simulink model "model_T_PSH_IEEE39"  (R2020b)
settings: Solver=ode3  StartTime=0.0  StopTime=300  FixedStep=Ts  RelTol=1e-3
PostLoadFcn:
  | IEEE39BusLineLength;
  | vNomHV = 345E3;fNom=60;load('Dynamicload.mat');
InitFcn:
  | IEEE39BusLineLength;
  | vNomHV = 345E3;fNom=60;load('Dynamicload.mat');
values from neighbouring files (symbols this model uses):
  At = 1.48    [MAIN_T_PSH_IEEE39.m]
  Dturb = 0.3    [MAIN_T_PSH_IEEE39.m]
  fix_mode = 1    [MAIN_T_PSH_IEEE39.m]
  Gmax = 1    [MAIN_T_PSH_IEEE39.m]
  Gmin = 0    [MAIN_T_PSH_IEEE39.m]
  Hdam = 1    [MAIN_T_PSH_IEEE39.m]
  Kd = 1    [MAIN_T_PSH_IEEE39.m]    (also in plots_T_PSH_IEEE39.m)
  max_delay_gen2pump = 20    [MAIN_T_PSH_IEEE39.m]
  max_delay_pump2hsc = 30    [MAIN_T_PSH_IEEE39.m]
  pgen_pump = Kd*Pref    (= 0.9)    [MAIN_T_PSH_IEEE39.m]
  pgen_turb = (1-Kd)*Pref    (= 0)    [MAIN_T_PSH_IEEE39.m]
  pgen_turb_gen2pump = (1-kd_gen2pump)*Pref    (= 0)    [MAIN_T_PSH_IEEE39.m]
  pgen_turb_hsc2gen = (1-kd_hsc2gen)*Pref    (= 0.36)    [MAIN_T_PSH_IEEE39.m]
  pgen_turb_pump2hsc = (1-kd_pump2hsc)*Pref    (= 0.36)    [MAIN_T_PSH_IEEE39.m]
  Pref = 0.9    [MAIN_T_PSH_IEEE39.m]    (also in MAIN_VS_PSH.m = 1)
  qNL = 0.1    [MAIN_T_PSH_IEEE39.m]
  R = 0.04    [MAIN_T_PSH_IEEE39.m]
  r = 0.31    [MAIN_T_PSH_IEEE39.m]
  Rp = 0.05    [IEEE39BusLineLength.m]
  Sn = 320E6    (= 320000000)    [MAIN_T_PSH_IEEE39.m]
  t_gen2pump = 10    [MAIN_T_PSH_IEEE39.m]
  t_hsc2gen = 150    [MAIN_T_PSH_IEEE39.m]
  t_pump2hsc = 35    [MAIN_T_PSH_IEEE39.m]
  t_sw_off = 220    [MAIN_FS_PSH_IEEE39.m]    (also in MAIN_T_PSH_IEEE39.m; MAIN_VS_PSH.m = 45)
  t_sw_on = 130    [MAIN_FS_PSH_IEEE39.m]    (also in MAIN_T_PSH_IEEE39.m; MAIN_VS_PSH.m = 35)
  Tf = 0.05    [MAIN_T_PSH_IEEE39.m]
  Tg = 0.5    [MAIN_T_PSH_IEEE39.m]
  TL_10_11_len = 14    [IEEE39BusLineLength.m]
  TL_10_13_len = 14    [IEEE39BusLineLength.m]
  TL_13_14_len = 32    [IEEE39BusLineLength.m]
  TL_14_15_len = 70    [IEEE39BusLineLength.m]
  TL_15_16_len = 31.5    [IEEE39BusLineLength.m]
  TL_16_17_len = 26    [IEEE39BusLineLength.m]
  TL_16_19_len = 61    [IEEE39BusLineLength.m]
  TL_16_21_len = 46    [IEEE39BusLineLength.m]
  TL_16_24_len = 15    [IEEE39BusLineLength.m]
  TL_17_18_len = 26    [IEEE39BusLineLength.m]
  TL_17_27_len = 59    [IEEE39BusLineLength.m]
  TL_1_2_len = 134    [IEEE39BusLineLength.m]
  TL_1_39_len = 105    [IEEE39BusLineLength.m]
  TL_21_22_len = 47    [IEEE39BusLineLength.m]
  TL_22_23_len = 33    [IEEE39BusLineLength.m]
  TL_24_23_len = 88    [IEEE39BusLineLength.m]
  TL_25_26_len = 101    [IEEE39BusLineLength.m]
  TL_26_27_len = 46.5    [IEEE39BusLineLength.m]
  TL_26_28_len = 151    [IEEE39BusLineLength.m]
  TL_26_29_len = 200    [IEEE39BusLineLength.m]
  TL_28_29_len = 48    [IEEE39BusLineLength.m]
  TL_2_25_len = 28    [IEEE39BusLineLength.m]
  TL_2_2_len = 49    [IEEE39BusLineLength.m]
  TL_3_18_len = 42    [IEEE39BusLineLength.m]
  TL_3_4_len = 53    [IEEE39BusLineLength.m]
  TL_4_14_len = 33    [IEEE39BusLineLength.m]
  TL_4_5_len = 32.5    [IEEE39BusLineLength.m]
  TL_5_6_len = 14    [IEEE39BusLineLength.m]
  TL_5_8_len = 32    [IEEE39BusLineLength.m]
  TL_6_11_len = 26.5    [IEEE39BusLineLength.m]
  TL_6_7_len = 25.5    [IEEE39BusLineLength.m]
  TL_7_8_len = 15    [IEEE39BusLineLength.m]
  TL_8_9_len = 93    [IEEE39BusLineLength.m]
  TL_9_39_len = 136    [IEEE39BusLineLength.m]
  Tr = 6.88    [MAIN_T_PSH_IEEE39.m]
  Ts = 25e-6    (= 2.5e-05)    [MAIN_FS_PSH_IEEE39.m]    (also in MAIN_T_PSH_IEEE39.m; MAIN_VS_PSH.m = 1e-07)
  Velm = 0.05    [MAIN_T_PSH_IEEE39.m]
  Vn = 18000    [MAIN_T_PSH_IEEE39.m]
undefined symbols (not defined in the file or in its folder): D1, Delta, load15, load16, load18, load20, load21, load23, load24, load25, load26, load27, load28, load29, load3, load39, load4, load7, load8
libraries: powerlib x216, sps_avr x10, simulink_extras x7, powerlib_meascontrol x5, simulink x1
(part 7 of 9)

== system model_T_PSH_IEEE39/SS_NorthSystem1/GT 8 ==
  5 MW : powerlib/Elements/Three-Phase Parallel RLC Load  LConnTagsString=A|B|C  Configuration=Y (grounded)  NominalVoltage=22e3  Vabc=[1e3 1e3 1e3]  Vabcp=[1e3 1e3 1e3]  NominalFrequency=fNom  UnbalancedPower=off  ActivePower=5e6  InductivePower=0  CapacitivePower=0  Pabc=[10e3 9e3 11e3]  QLabc=[100 90 110]  QCabc=[100 90 110]  Pabcp=[10e3 9e3 11e3]  QLabcp=[100 90 110]  QCabcp=[100 90 110]  Measurements=None  LoadType=constant Z
  Bus Selector1 : BusSelector  OutputSignals="dq0 components.Stator voltage  vq (pu),dq0 components.Stator voltage  vd (pu),Mechanical.Rotor speed  wm  (pu),Mechanical.Rotor speed deviation  dw (pu),Output active power   Peo (pu),Output reactive power  Qeo (pu)"
  Bus 37 : powerlib/Measurements/Three-Phase V-I Measurement  VoltageMeasurement=phase-to-ground  SetLabelV=on  LabelV=V_bus_G8  Vpu=off  VpuLL=off  CurrentMeasurement=no  SetLabelI=on  LabelI=I_bus_G8  Ipu=off  Pbase=100e6  Vbase=16.5e3  OutputType=Complex  PhasorSimulation=off  PSBequivalent=0
  Excitation System : sps_avr/Excitation System  tr=20e-3  reg=[ 200, 0.02 ]  exc=[ 1, 0 .19]  tgr=[ 0, 0 ]  damp=[ 0.0012, 1 ]  sat=[ 0, 0 ]  lim=[ 0, 7.32, 0 ]  v0=[1.01 1.6849]
      settings: SourceProductBaseCode=PS
  GT1_CB11 : Subsystem
  Ground : Ground
  HTG : powerlib/Machines/Hydraulic Turbine and Governor  sm="[ 10/3  0.07 ]"  gate="[  0.01  0.97518  -0.1  0.1 ]"  reg="[  Rp  1.163  0.105  0  0.01  ]"  hyd="[  0  2.67  ]"  dref=0  po=0.6
      settings: SourceProductBaseCode=PS
  Load Flow Bus : powerlib/Measurements/Load Flow Bus  LConnTagsString=a  Phases=single  Connectors=on one side  ID=Bus-37  Vbase=22000  Vref=1.01  Vangle=0  VLF=1.01  VLFb=1  VLFc=1  angleLF=3.342  angleLFb=0  angleLFc=0
      settings: AttributesFormatString=%<ID>\n%<Vbase>V\n%<VLF>pu\n%<angleLF>deg.
  Machine 8 1000 MVA 22 kV : powerlib/Machines/Synchronous Machine pu Standard  PresetModel=No  MechanicalLoad=Mechanical power Pm  ShowDetailedParameters=on  RotorType=Round  Units=per unit standard parameters  MeasurementBus=off  NominalParameters="[ 1000E6  22000   fNom]"  Reactances1=[ 2.035 0.4 0.2 1.965 0.639 0.2 0.028 ]  Reactances2=[ 0.995, 0.195, 0.155, 0.568, 0.143, 0.16 ]  dAxisTimeConstants=Open-circuit  qAxisTimeConstants=Open-circuit  TimeConstants1=[]  TimeConstants2=[6.7 0.03 0.41 0.04]  TimeConstants3=[]  TimeConstants4=[]  TimeConstants5=[ 9.2, 0.01, 0.01 ]  TimeConstants6=[]  TimeConstants7=[]  TimeConstants8=[]  StatorResistance=0.005  Mechanical=[ 3.46 0.02 20]  PolePairs=20  InitialConditions=[0 -37.6671 0.634647 0.634647 0.634647 0.151083 -119.849 120.151 1.68493]  SetSaturation=off  Saturation=[0.6404,0.7127,0.8441,0.9214,0.9956,1.082,1.19,1.316,1.457;0.7,0.7698,0.8872,0.9466,0.9969,1.046,1.1,1.151,1.201]  LoadFlowParameters=[1 540000000 22611.6 0]  TsPowergui=0  TsBlock=-1  IterativeModel=Trapezoidal non iterative  IterativeDiscreteModel=Trapezoidal non iterative  BusType=PV  Pref=6.4e+008  Qref=0  Qmin=-500e6  Qmax=50e6  PLF=0  QLF=0
      settings: AttributesFormatString=\n\n
  Pref : Constant  Value=0.6
  Terminator5 : Terminator
  Transformer 8 772.2 MVA 22 kV / 345 kV : powerlib/Elements/Three-Phase Transformer (Two Windings)  Winding1Connection=Delta (D1)  Winding2Connection=Yg  CoreType=Three single-phase transformers  SetSaturation=off  Hysteresis=off  DataFile='hysteresis'  SetInitialFlux=off  Measurements=None  UNITS=pu  NominalPower=[ 1000e6 fNom]  Winding1="[ 22e3    0.0006*1000/100/2  0.0232*1000/100/2 ]"  Winding2="[ 1.025*345e3    0.0006*1000/100/2  0.0232*1000/100/2  ]"  Rm=500  Lm=500  L0=0.5  Saturation="[ 0,0  ;  0.005,1.2  ;  1.0,1.4 ]"  InitialFluxes=[ 0.8 , -0.8 , 0.7 ]  BreakLoop=off  DiscreteSolver=Trapezoidal iterative  DataType=off  TransfoNumber=0
  Vref : Constant  Value=1.01
  wref : Constant
  A : PMIOPort  Side=Right
  B : PMIOPort  Port=2  Side=Right
  C : PMIOPort  Port=3  Side=Right
  tag scope: P_G8=global, Q_G8=global, V_G8=global, Wm_G8=global
  wires:
  [V_bus_G8] -> [V_G8]
  Bus Selector1/6 -> [Q_G8]  "<Output reactive power  Qeo (pu)>"
  Bus Selector1/5 -> [P_G8], HTG/4  "<Output active power   Peo (pu)>"
  Bus Selector1/4 -> HTG/5  "<Rotor speed deviation  dw (pu)>"
  Bus Selector1/3 -> [Wm_G8], HTG/3  "<Rotor speed  wm  (pu)>"
  Bus Selector1/2 -> Excitation System/2  "<Stator voltage  vd (pu)>"
  Bus Selector1/1 -> Excitation System/3  "<Stator voltage  vq (pu)>"
  Machine 8 1000 MVA 22 kV/1 -> Bus Selector1/1
  HTG/1 -> Machine 8 1000 MVA 22 kV/1
  Excitation System/1 -> Machine 8 1000 MVA 22 kV/2
  wref/1 -> HTG/1
  Pref/1 -> HTG/2
  Vref/1 -> Excitation System/1
  HTG/2 -> Terminator5/1
  Ground/1 -> Excitation System/4
  connections:
  Machine 8 1000 MVA 22 kV/RConn3 -- Bus 37/LConn3
  Machine 8 1000 MVA 22 kV/RConn2 -- Bus 37/LConn2
  Machine 8 1000 MVA 22 kV/RConn1 -- Bus 37/LConn1
  5 MW/LConn3 -- Bus 37/RConn3 -- Transformer 8 772.2 MVA 22 kV / 345 kV/LConn3
  5 MW/LConn2 -- Bus 37/RConn2 -- Transformer 8 772.2 MVA 22 kV / 345 kV/LConn2
  5 MW/LConn1 -- Bus 37/RConn1 -- Load Flow Bus/LConn1 -- Transformer 8 772.2 MVA 22 kV / 345 kV/LConn1
  GT1_CB11/LConn1 -- Transformer 8 772.2 MVA 22 kV / 345 kV/RConn1
  GT1_CB11/LConn2 -- Transformer 8 772.2 MVA 22 kV / 345 kV/RConn2
  GT1_CB11/LConn3 -- Transformer 8 772.2 MVA 22 kV / 345 kV/RConn3
  C/RConn1 -- GT1_CB11/RConn3
  B/RConn1 -- GT1_CB11/RConn2
  A/RConn1 -- GT1_CB11/RConn1

== system model_T_PSH_IEEE39/SS_NorthSystem1/GT 9 ==
  5 MW : powerlib/Elements/Three-Phase Parallel RLC Load  LConnTagsString=A|B|C  Configuration=Y (grounded)  NominalVoltage=22e3  Vabc=[1e3 1e3 1e3]  Vabcp=[1e3 1e3 1e3]  NominalFrequency=fNom  UnbalancedPower=off  ActivePower=5e6  InductivePower=0  CapacitivePower=0  Pabc=[10e3 9e3 11e3]  QLabc=[100 90 110]  QCabc=[100 90 110]  Pabcp=[10e3 9e3 11e3]  QLabcp=[100 90 110]  QCabcp=[100 90 110]  Measurements=None  LoadType=constant Z
  Bus Selector1 : BusSelector  OutputSignals="dq0 components.Stator voltage  vq (pu),dq0 components.Stator voltage  vd (pu),Mechanical.Rotor speed  wm  (pu),Mechanical.Rotor speed deviation  dw (pu),Output active power   Peo (pu),Output reactive power  Qeo (pu)"
  Bus 38 : powerlib/Measurements/Three-Phase V-I Measurement  VoltageMeasurement=phase-to-ground  SetLabelV=on  LabelV=V_bus_G9  Vpu=off  VpuLL=off  CurrentMeasurement=no  SetLabelI=on  LabelI=I_bus_G9  Ipu=off  Pbase=100e6  Vbase=16.5e3  OutputType=Complex  PhasorSimulation=off  PSBequivalent=0
  Excitation System : sps_avr/Excitation System  tr=20e-3  reg=[ 200, 0.02 ]  exc=[ 1, 0 .19]  tgr=[ 0, 0 ]  damp=[ 0.0012, 1 ]  sat=[ 0, 0 ]  lim=[ 0, 7.32, 0 ]  v0=[1.0156 1.6973]
      settings: SourceProductBaseCode=PS
  GT1_CB12 : Subsystem
  Ground : Ground
  HTG : powerlib/Machines/Hydraulic Turbine and Governor  sm="[ 10/3  0.07 ]"  gate="[  0.01  0.97518  -0.1  0.1 ]"  reg="[  Rp  1.163  0.105  0  0.01  ]"  hyd="[  0  2.67  ]"  dref=0  po=0.654
      settings: SourceProductBaseCode=PS
  Load Flow Bus : powerlib/Measurements/Load Flow Bus  LConnTagsString=a  Phases=single  Connectors=on one side  ID=Bus-38  Vbase=22000  Vref=1.0265  Vangle=0  VLF=1.016  VLFb=1  VLFc=1  angleLF=1.986  angleLFb=0  angleLFc=0
      settings: AttributesFormatString=%<ID>\n%<Vbase>V\n%<VLF>pu\n%<angleLF>deg.
  Machine 9 1000 MVA 22 kV : powerlib/Machines/Synchronous Machine pu Standard  PresetModel=No  MechanicalLoad=Mechanical power Pm  ShowDetailedParameters=on  RotorType=Round  Units=per unit standard parameters  MeasurementBus=off  NominalParameters="[ 1000E6  22000   fNom]"  Reactances1=[ 1.7901 0.4845 0.242 1.742 0.4989 0.242 0.03 ]  Reactances2=[ 0.995, 0.195, 0.155, 0.568, 0.143, 0.16 ]  dAxisTimeConstants=Open-circuit  qAxisTimeConstants=Open-circuit  TimeConstants1=[]  TimeConstants2=[4.79 0.03 1.96 0.04]  TimeConstants3=[]  TimeConstants4=[]  TimeConstants5=[ 9.2, 0.01, 0.01 ]  TimeConstants6=[]  TimeConstants7=[]  TimeConstants8=[]  StatorResistance=0.005  Mechanical=[ 4.058 0.02 20]  PolePairs=20  InitialConditions=[0 -39.4462 0.720476 0.720476 0.720476 -1.93203 -121.932 118.068 1.69726]  SetSaturation=off  Saturation=[0.6404,0.7127,0.8441,0.9214,0.9956,1.082,1.19,1.316,1.457;0.7,0.7698,0.8872,0.9466,0.9969,1.046,1.1,1.151,1.201]  LoadFlowParameters=[1 830000000 22583 0]  TsPowergui=0  TsBlock=-1  IterativeModel=Trapezoidal non iterative  IterativeDiscreteModel=Trapezoidal non iterative  BusType=PV  Pref=7.3e+008  Qref=0  Qmin=-500e6  Qmax=50e6  PLF=0  QLF=0
      settings: AttributesFormatString=\n\n
  Terminator5 : Terminator
  Transformer 9 935 MVA 22 kV / 345 kV : powerlib/Elements/Three-Phase Transformer (Two Windings)  Winding1Connection=Delta (D1)  Winding2Connection=Yg  CoreType=Three single-phase transformers  SetSaturation=off  Hysteresis=off  DataFile='hysteresis'  SetInitialFlux=off  Measurements=None  UNITS=pu  NominalPower=[ 935e6 fNom]  Winding1="[ 22e3  0.0008*935/100/2  0.0156*935/100/2]"  Winding2="[ 1.025*345e3  0.0008*935/100/2  0.0156*935/100/2]"  Rm=500  Lm=500  L0=0.5  Saturation="[ 0,0  ;  0.005,1.2  ;  1.0,1.4 ]"  InitialFluxes=[ 0.8 , -0.8 , 0.7 ]  BreakLoop=off  DiscreteSolver=Trapezoidal iterative  DataType=off  TransfoNumber=0
  wref : Constant
  wref1 : Constant  Value=0.654
  wref2 : Constant  Value=1.0265
  A : PMIOPort  Side=Right
  B : PMIOPort  Port=2  Side=Right
  C : PMIOPort  Port=3  Side=Right
  tag scope: P_G9=global, Q_G9=global, V_G9=global, Wm_G9=global
  wires:
  Ground/1 -> Excitation System/4
  HTG/2 -> Terminator5/1
  wref2/1 -> Excitation System/1
  wref1/1 -> HTG/2
  wref/1 -> HTG/1
  Excitation System/1 -> Machine 9 1000 MVA 22 kV/2
  HTG/1 -> Machine 9 1000 MVA 22 kV/1
  Machine 9 1000 MVA 22 kV/1 -> Bus Selector1/1
  Bus Selector1/1 -> Excitation System/3  "<Stator voltage  vq (pu)>"
  Bus Selector1/2 -> Excitation System/2  "<Stator voltage  vd (pu)>"
  Bus Selector1/3 -> HTG/3, [Wm_G9]  "<Rotor speed  wm  (pu)>"
  Bus Selector1/4 -> HTG/5  "<Rotor speed deviation  dw (pu)>"
  Bus Selector1/5 -> HTG/4, [P_G9]  "<Output active power   Peo (pu)>"
  Bus Selector1/6 -> [Q_G9]  "<Output reactive power  Qeo (pu)>"
  [V_bus_G9] -> [V_G9]
  connections:
  Transformer 9 935 MVA 22 kV / 345 kV/LConn1 -- Load Flow Bus/LConn1 -- Bus 38/RConn1 -- 5 MW/LConn1
  Transformer 9 935 MVA 22 kV / 345 kV/LConn2 -- Bus 38/RConn2 -- 5 MW/LConn2
  Transformer 9 935 MVA 22 kV / 345 kV/LConn3 -- Bus 38/RConn3 -- 5 MW/LConn3
  Machine 9 1000 MVA 22 kV/RConn1 -- Bus 38/LConn1
  Machine 9 1000 MVA 22 kV/RConn2 -- Bus 38/LConn2
  Machine 9 1000 MVA 22 kV/RConn3 -- Bus 38/LConn3
  Transformer 9 935 MVA 22 kV / 345 kV/RConn2 -- GT1_CB12/LConn2
  Transformer 9 935 MVA 22 kV / 345 kV/RConn1 -- GT1_CB12/LConn1
  Transformer 9 935 MVA 22 kV / 345 kV/RConn3 -- GT1_CB12/LConn3
  B/RConn1 -- GT1_CB12/RConn2
  C/RConn1 -- GT1_CB12/RConn3
  A/RConn1 -- GT1_CB12/RConn1

== system model_T_PSH_IEEE39/SS_NorthSystem1/Load 25 ==
  Terminator : Terminator
  Three-Phase Dynamic Load : powerlib/Elements/Three-Phase Dynamic Load  NominalVoltage="[345e3  fNom]"  ActiveReactivePowers=[2.24e+08 4.72e+07]  PositiveSequence=[1.03404 25.0543]  ExternalControl=on  NpNq=[0 0]  TimeConstants="[0  0  0  0]"  MinimumVoltage=0.7  Tfilter=1e-4  LoadFlowParameters=[4,0,0,0,0]
      settings: SourceProductBaseCode=PS
  V_Bus_L25 : powerlib/Measurements/Three-Phase V-I Measurement  VoltageMeasurement=phase-to-ground  SetLabelV=off  LabelV=V_Bus_L25  Vpu=off  VpuLL=off  CurrentMeasurement=yes  SetLabelI=on  LabelI=I_L25  Ipu=off  Pbase=100e6  Vbase=230e3  OutputType=Complex  PhasorSimulation=off  PSBequivalent=0
  A : PMIOPort  Side=Left
  B : PMIOPort  Port=2  Side=Left
  C : PMIOPort  Port=3  Side=Left
  tag scope: V_L25=global
  wires:
  Three-Phase Dynamic Load/1 -> Terminator/1
  V_Bus_L25/1 -> [V_L25]
  [load25] -> Three-Phase Dynamic Load/1
  connections:
  V_Bus_L25/RConn1 -- Three-Phase Dynamic Load/LConn1
  C/RConn1 -- V_Bus_L25/LConn3
  B/RConn1 -- V_Bus_L25/LConn2
  A/RConn1 -- V_Bus_L25/LConn1
  V_Bus_L25/RConn2 -- Three-Phase Dynamic Load/LConn2
  V_Bus_L25/RConn3 -- Three-Phase Dynamic Load/LConn3

== system model_T_PSH_IEEE39/SS_NorthSystem1/Load 26 ==
  Bus_L26 : powerlib/Measurements/Three-Phase V-I Measurement  VoltageMeasurement=phase-to-ground  SetLabelV=off  LabelV=V_Bus_L26  Vpu=off  VpuLL=off  CurrentMeasurement=yes  SetLabelI=on  LabelI=I_L26  Ipu=off  Pbase=100e6  Vbase=230e3  OutputType=Complex  PhasorSimulation=off  PSBequivalent=0
  Terminator : Terminator
  Three-Phase Dynamic Load : powerlib/Elements/Three-Phase Dynamic Load  NominalVoltage=[345e3 fNom]  ActiveReactivePowers=[1.39e+08 1.7e+07]  PositiveSequence=[1.02673 21.7857]  ExternalControl=on  NpNq=[0 0]  TimeConstants="[0  0  0  0]"  MinimumVoltage=0.7  Tfilter=1e-4  LoadFlowParameters=[4,0,0,0,0]
      settings: SourceProductBaseCode=PS
  A : PMIOPort  Side=Left
  B : PMIOPort  Port=2  Side=Left
  C : PMIOPort  Port=3  Side=Left
  tag scope: V_L26=global
  wires:
  Three-Phase Dynamic Load/1 -> Terminator/1
  Bus_L26/1 -> [V_L26]
  [load26] -> Three-Phase Dynamic Load/1
  connections:
  Three-Phase Dynamic Load/LConn1 -- Bus_L26/RConn1
  C/RConn1 -- Bus_L26/LConn3
  B/RConn1 -- Bus_L26/LConn2
  A/RConn1 -- Bus_L26/LConn1
  Bus_L26/RConn2 -- Three-Phase Dynamic Load/LConn2
  Bus_L26/RConn3 -- Three-Phase Dynamic Load/LConn3

== system model_T_PSH_IEEE39/SS_NorthSystem1/Load 28 ==
  Bus_L28 : powerlib/Measurements/Three-Phase V-I Measurement  VoltageMeasurement=phase-to-ground  SetLabelV=off  LabelV=V_Bus_L28  Vpu=off  VpuLL=off  CurrentMeasurement=yes  SetLabelI=on  LabelI=I_L28  Ipu=off  Pbase=100e6  Vbase=230e3  OutputType=Complex  PhasorSimulation=off  PSBequivalent=0
  Terminator : Terminator
  Three-Phase Dynamic Load : powerlib/Elements/Three-Phase Dynamic Load  NominalVoltage=[345e3 fNom]  ActiveReactivePowers=[2.06e+08 2.76e+07]  PositiveSequence=[1.03092 23.6623]  ExternalControl=on  NpNq=[0 0]  TimeConstants="[0  0  0  0]"  MinimumVoltage=0.7  Tfilter=1e-4  LoadFlowParameters=[4,0,0,0,0]
      settings: SourceProductBaseCode=PS
  A : PMIOPort  Side=Left
  B : PMIOPort  Port=2  Side=Left
  C : PMIOPort  Port=3  Side=Left
  tag scope: V_L28=global
  wires:
  Three-Phase Dynamic Load/1 -> Terminator/1
  Bus_L28/1 -> [V_L28]
  [load28] -> Three-Phase Dynamic Load/1
  connections:
  Bus_L28/RConn3 -- Three-Phase Dynamic Load/LConn3
  Bus_L28/RConn2 -- Three-Phase Dynamic Load/LConn2
  A/RConn1 -- Bus_L28/LConn1
  B/RConn1 -- Bus_L28/LConn2
  C/RConn1 -- Bus_L28/LConn3
  Bus_L28/RConn1 -- Three-Phase Dynamic Load/LConn1

== system model_T_PSH_IEEE39/SS_NorthSystem1/Load 29 ==
  Bus_L29 : powerlib/Measurements/Three-Phase V-I Measurement  VoltageMeasurement=phase-to-ground  SetLabelV=off  LabelV=V_Bus_L29  Vpu=off  VpuLL=off  CurrentMeasurement=yes  SetLabelI=on  LabelI=I_L29  Ipu=off  Pbase=100e6  Vbase=230e3  OutputType=Complex  PhasorSimulation=off  PSBequivalent=0
  Terminator : Terminator
  Three-Phase Dynamic Load : powerlib/Elements/Three-Phase Dynamic Load  NominalVoltage=[345e3 fNom]  ActiveReactivePowers=[2.835e+08 2.69e+07]  PositiveSequence=[1.03368 25.6776]  ExternalControl=on  NpNq=[0 0]  TimeConstants="[0  0  0  0]"  MinimumVoltage=0.7  Tfilter=1e-4  LoadFlowParameters=[4,0,0,0,0]
      settings: SourceProductBaseCode=PS
  A : PMIOPort  Side=Left
  B : PMIOPort  Port=2  Side=Left
  C : PMIOPort  Port=3  Side=Left
  tag scope: V_L29=global
  wires:
  Three-Phase Dynamic Load/1 -> Terminator/1
  Bus_L29/1 -> [V_L29]
  [load29] -> Three-Phase Dynamic Load/1
  connections:
  Three-Phase Dynamic Load/LConn1 -- Bus_L29/RConn1
  C/RConn1 -- Bus_L29/LConn3
  B/RConn1 -- Bus_L29/LConn2
  A/RConn1 -- Bus_L29/LConn1
  Bus_L29/RConn2 -- Three-Phase Dynamic Load/LConn2
  Bus_L29/RConn3 -- Three-Phase Dynamic Load/LConn3

== system model_T_PSH_IEEE39/SS_NorthSystem1/Machines Measurements ==
  Mux : Mux  Inputs=2
  Mux1 : Mux
  Mux2 : Mux
  Machines Measurements : Outport
  wires:
  Mux2/1 -> Mux/2
  Mux1/1 -> Mux/1
  Mux/1 -> Machines Measurements/1
  [Wm_G9] -> Mux2/4
  [Q_G9] -> Mux2/3
  [P_G9] -> Mux2/2
  [V_G9] -> Mux2/1
  [Wm_G8] -> Mux1/4
  [Q_G8] -> Mux1/3
  [P_G8] -> Mux1/2
  [V_G8] -> Mux1/1

== system model_T_PSH_IEEE39/SS_NorthSystem2/Buses current_N ==
  Mux3 : Mux  Inputs=6
  curremt : Outport
  wires:
  [I_bus_1] -> Mux3/1
  [I_bus_2] -> Mux3/2
  [I_L3] -> Mux3/3
  [I_bus_17] -> Mux3/4
  [I_L18] -> Mux3/5
  Mux3/1 -> curremt/1
  [I_L27] -> Mux3/6

== system model_T_PSH_IEEE39/SS_NorthSystem2/Buses voltages_N ==
  Mux3 : Mux  Inputs=6
  Voltages : Outport
  wires:
  Mux3/1 -> Voltages/1
  [V_L27] -> Mux3/6
  [V_L18] -> Mux3/5
  [V_bus_17] -> Mux3/4
  [V_L3] -> Mux3/3
  [V_bus_2] -> Mux3/2
  [V_bus_1] -> Mux3/1

== system model_T_PSH_IEEE39/SS_NorthSystem2/GT 10 ==
  5 MW : powerlib/Elements/Three-Phase Parallel RLC Load  LConnTagsString=A|B|C  Configuration=Y (grounded)  NominalVoltage=22e3  Vabc=[1e3 1e3 1e3]  Vabcp=[1e3 1e3 1e3]  NominalFrequency=fNom  UnbalancedPower=off  ActivePower=5e6  InductivePower=0  CapacitivePower=0  Pabc=[10e3 9e3 11e3]  QLabc=[100 90 110]  QCabc=[100 90 110]  Pabcp=[10e3 9e3 11e3]  QLabcp=[100 90 110]  QCabcp=[100 90 110]  Measurements=None  LoadType=constant Z
  Bus Selector1 : BusSelector  OutputSignals="dq0 components.Stator voltage  vq (pu),dq0 components.Stator voltage  vd (pu),Mechanical.Rotor speed  wm  (pu),Mechanical.Rotor speed deviation  dw (pu),Output active power   Peo (pu),Output reactive power  Qeo (pu)"
  Bus 30 : powerlib/Measurements/Three-Phase V-I Measurement  VoltageMeasurement=phase-to-ground  SetLabelV=on  LabelV=V_bus_G10  Vpu=off  VpuLL=off  CurrentMeasurement=no  SetLabelI=on  LabelI=I_bus_G10  Ipu=off  Pbase=100e6  Vbase=16.5e3  OutputType=Complex  PhasorSimulation=off  PSBequivalent=0
  Excitation System : sps_avr/Excitation System  tr=20e-3  reg=[ 200, 0.02 ]  exc=[ 1, 0 .19]  tgr=[ 0, 0 ]  damp=[ 0.0012, 1 ]  sat=[ 0, 0 ]  lim=[ 0, 7.32, 0 ]  v0=[1.025 1.2732]
      settings: SourceProductBaseCode=PS
  GT1_CB14 : Subsystem
  Ground : Ground
  HTG : powerlib/Machines/Hydraulic Turbine and Governor  sm="[ 10/3  0.07 ]"  gate="[  0.01  0.97518  -0.1  0.1 ]"  reg="[  Rp  1.163  0.105  0  0.01  ]"  hyd="[  0  2.67  ]"  dref=0  po=0.324
      settings: SourceProductBaseCode=PS
  Load Flow Bus : powerlib/Measurements/Load Flow Bus  LConnTagsString=a  Phases=single  Connectors=on one side  ID=Bus-30  Vbase=22000  Vref=1.025  Vangle=0  VLF=1.025  VLFb=1  VLFc=1  angleLF=-2.488  angleLFb=0  angleLFc=0
      settings: AttributesFormatString=%<ID>\n%<Vbase>V\n%<VLF>pu\n%<angleLF>deg.
  Machine 10 1000 MVA 22 kV : powerlib/Machines/Synchronous Machine pu Standard  PresetModel=No  MechanicalLoad=Mechanical power Pm  ShowDetailedParameters=on  RotorType=Round  Units=per unit standard parameters  MeasurementBus=off  NominalParameters="[ 1000E6  22000   fNom]"  Reactances1="[ 1.29 0.4 0.2 0.89 0.103 0.2 0.013  ]"  Reactances2=[ 0.995, 0.195, 0.155, 0.568, 0.143, 0.16 ]  dAxisTimeConstants=Open-circuit  qAxisTimeConstants=Open-circuit  TimeConstants1=[]  TimeConstants2=[10.2 0.03 0.02 0.04]  TimeConstants3=[]  TimeConstants4=[]  TimeConstants5=[ 9.2, 0.01, 0.01 ]  TimeConstants6=[]  TimeConstants7=[]  TimeConstants8=[]  StatorResistance=0.005  Mechanical=[ 3.255 0.02 20]  PolePairs=20  InitialConditions=[0 -77.6756 0.367118 0.367118 0.367118 -24.0341 -144.034 95.9659 1.27317]  SetSaturation=off  Saturation=[0.6404,0.7127,0.8441,0.9214,0.9956,1.082,1.19,1.316,1.457;0.7,0.7698,0.8872,0.9466,0.9969,1.046,1.1,1.151,1.201]  LoadFlowParameters=[1 632000000 21938.4 0]  TsPowergui=0  TsBlock=-1  IterativeModel=Trapezoidal non iterative  IterativeDiscreteModel=Trapezoidal non iterative  BusType=PV  Pref=3.5e+008  Qref=0  Qmin=-500e6  Qmax=200e6  PLF=0  QLF=0
      settings: AttributesFormatString=\n\n
  Pref : Constant  Value=0.324
  Terminator5 : Terminator
  Transformer 10 1419 MVA 22 kV / 345 kV : powerlib/Elements/Three-Phase Transformer (Two Windings)  Winding1Connection=Delta (D1)  Winding2Connection=Yg  CoreType=Three single-phase transformers  SetSaturation=off  Hysteresis=off  DataFile='hysteresis'  SetInitialFlux=off  Measurements=None  UNITS=pu  NominalPower=[ 1419e6 fNom]  Winding1="[ 22e3   0    0.0181*1419/100/2 ]"  Winding2=|  Rm=500  Lm=500  L0=0.5  Saturation="[ 0,0  ;  0.005,1.2  ;  1.0,1.4 ]"  InitialFluxes=[ 0.8 , -0.8 , 0.7 ]  BreakLoop=off  DiscreteSolver=Trapezoidal iterative  DataType=off  TransfoNumber=0
      | [ 1.025*345e3 0    0.0181*1419/100/2
      | ]
  Vref : Constant  Value=1.025
  wref : Constant
  A : PMIOPort  Side=Right
  B : PMIOPort  Port=2  Side=Right
  C : PMIOPort  Port=3  Side=Right
  tag scope: P_G10=global, Q_G10=global, V_G10=global, Wm_G10=global
  wires:
  Ground/1 -> Excitation System/4
  HTG/2 -> Terminator5/1
  Vref/1 -> Excitation System/1
  Pref/1 -> HTG/2
  wref/1 -> HTG/1
  Excitation System/1 -> Machine 10 1000 MVA 22 kV/2
  HTG/1 -> Machine 10 1000 MVA 22 kV/1
  Machine 10 1000 MVA 22 kV/1 -> Bus Selector1/1
  Bus Selector1/1 -> Excitation System/3  "<Stator voltage  vq (pu)>"
  Bus Selector1/2 -> Excitation System/2  "<Stator voltage  vd (pu)>"
  Bus Selector1/3 -> HTG/3, [Wm_G10]  "<Rotor speed  wm  (pu)>"
  Bus Selector1/4 -> HTG/5  "<Rotor speed deviation  dw (pu)>"
  Bus Selector1/5 -> HTG/4, [P_G10]  "<Output active power   Peo (pu)>"
  Bus Selector1/6 -> [Q_G10]  "<Output reactive power  Qeo (pu)>"
  [V_bus_G10] -> [V_G10]
  connections:
  Transformer 10 1419 MVA 22 kV / 345 kV/LConn1 -- Load Flow Bus/LConn1 -- Bus 30/RConn1 -- 5 MW/LConn1
  Transformer 10 1419 MVA 22 kV / 345 kV/LConn2 -- Bus 30/RConn2 -- 5 MW/LConn2
  Transformer 10 1419 MVA 22 kV / 345 kV/LConn3 -- Bus 30/RConn3 -- 5 MW/LConn3
  Machine 10 1000 MVA 22 kV/RConn1 -- Bus 30/LConn1
  Machine 10 1000 MVA 22 kV/RConn2 -- Bus 30/LConn2
  Machine 10 1000 MVA 22 kV/RConn3 -- Bus 30/LConn3
  GT1_CB14/LConn1 -- Transformer 10 1419 MVA 22 kV / 345 kV/RConn1
  GT1_CB14/LConn2 -- Transformer 10 1419 MVA 22 kV / 345 kV/RConn2
  GT1_CB14/LConn3 -- Transformer 10 1419 MVA 22 kV / 345 kV/RConn3
  A/RConn1 -- GT1_CB14/RConn1
  C/RConn1 -- GT1_CB14/RConn3
  B/RConn1 -- GT1_CB14/RConn2

== system model_T_PSH_IEEE39/SS_NorthSystem2/Load 18 ==
  Bus_L18 : powerlib/Measurements/Three-Phase V-I Measurement  VoltageMeasurement=phase-to-ground  SetLabelV=off  LabelV=V_Bus_L18  Vpu=off  VpuLL=off  CurrentMeasurement=yes  SetLabelI=on  LabelI=I_L18  Ipu=off  Pbase=100e6  Vbase=230e3  OutputType=Complex  PhasorSimulation=off  PSBequivalent=0
  Terminator : Terminator
  Three-Phase Dynamic Load : powerlib/Elements/Three-Phase Dynamic Load  NominalVoltage=[345e3 fNom]  ActiveReactivePowers=[1.58e+08 3e+07]  PositiveSequence=[1.0086 19.7218]  ExternalControl=on  NpNq=[0 0]  TimeConstants="[0  0  0  0]"  MinimumVoltage=0.7  Tfilter=1e-4  LoadFlowParameters=[4,0,0,0,0]
      settings: SourceProductBaseCode=PS
  A : PMIOPort  Side=Left
  B : PMIOPort  Port=2  Side=Left
  C : PMIOPort  Port=3  Side=Left
  tag scope: V_L18=global
  wires:
  Three-Phase Dynamic Load/1 -> Terminator/1
  Bus_L18/1 -> [V_L18]
  [load18] -> Three-Phase Dynamic Load/1
  connections:
  Bus_L18/RConn3 -- Three-Phase Dynamic Load/LConn3
  Bus_L18/RConn2 -- Three-Phase Dynamic Load/LConn2
  A/RConn1 -- Bus_L18/LConn1
  B/RConn1 -- Bus_L18/LConn2
  C/RConn1 -- Bus_L18/LConn3
  Bus_L18/RConn1 -- Three-Phase Dynamic Load/LConn1

== system model_T_PSH_IEEE39/SS_NorthSystem2/Load 27 ==
  Bus_L27 : powerlib/Measurements/Three-Phase V-I Measurement  VoltageMeasurement=phase-to-ground  SetLabelV=off  LabelV=V_Bus_L27  Vpu=off  VpuLL=off  CurrentMeasurement=yes  SetLabelI=on  LabelI=I_L27  Ipu=off  Pbase=100e6  Vbase=230e3  OutputType=Complex  PhasorSimulation=off  PSBequivalent=0
  Terminator : Terminator
  Three-Phase Dynamic Load : powerlib/Elements/Three-Phase Dynamic Load  NominalVoltage=[345e3 fNom]  ActiveReactivePowers=[2.81e+08 7.55e+07]  PositiveSequence=[1.0131 19.7618]  ExternalControl=on  NpNq=[0 0]  TimeConstants="[0  0  0  0]"  MinimumVoltage=0.7  Tfilter=1e-4  LoadFlowParameters=[4,0,0,0,0]
      settings: SourceProductBaseCode=PS
  A : PMIOPort  Side=Left
  B : PMIOPort  Port=2  Side=Left
  C : PMIOPort  Port=3  Side=Left
  tag scope: V_L27=global
  wires:
  Three-Phase Dynamic Load/1 -> Terminator/1
  Bus_L27/1 -> [V_L27]
  [load27] -> Three-Phase Dynamic Load/1
  connections:
  Bus_L27/RConn3 -- Three-Phase Dynamic Load/LConn3
  Bus_L27/RConn2 -- Three-Phase Dynamic Load/LConn2
  A/RConn1 -- Bus_L27/LConn1
  B/RConn1 -- Bus_L27/LConn2
  C/RConn1 -- Bus_L27/LConn3
  Three-Phase Dynamic Load/LConn1 -- Bus_L27/RConn1

== system model_T_PSH_IEEE39/SS_NorthSystem2/Load 3 ==
  Bus_L3 : powerlib/Measurements/Three-Phase V-I Measurement  VoltageMeasurement=phase-to-ground  SetLabelV=off  LabelV=V_Bus_L3  Vpu=off  VpuLL=off  CurrentMeasurement=yes  SetLabelI=on  LabelI=I_L3  Ipu=off  Pbase=100e6  Vbase=230e3  OutputType=Complex  PhasorSimulation=off  PSBequivalent=0
  Terminator : Terminator
  Three-Phase Dynamic Load : powerlib/Elements/Three-Phase Dynamic Load  NominalVoltage=[ 345e3 fNom]  ActiveReactivePowers=[5e+07 2.5e+07]  PositiveSequence=[1.01048 21.0012]  ExternalControl=on  NpNq=[0 0]  TimeConstants="[0  0  0  0]"  MinimumVoltage=0.7  Tfilter=1e-4  LoadFlowParameters=[4,0,0,0,0]
      settings: SourceProductBaseCode=PS
  A : PMIOPort  Side=Left
  B : PMIOPort  Port=2  Side=Left
  C : PMIOPort  Port=3  Side=Left
  tag scope: V_L3=global
  wires:
  Three-Phase Dynamic Load/1 -> Terminator/1
  Bus_L3/1 -> [V_L3]
  [load3] -> Three-Phase Dynamic Load/1
  connections:
  Bus_L3/RConn1 -- Three-Phase Dynamic Load/LConn1
  C/RConn1 -- Bus_L3/LConn3
  B/RConn1 -- Bus_L3/LConn2
  A/RConn1 -- Bus_L3/LConn1
  Bus_L3/RConn2 -- Three-Phase Dynamic Load/LConn2
  Bus_L3/RConn3 -- Three-Phase Dynamic Load/LConn3

== system model_T_PSH_IEEE39/SS_NorthSystem2/Machines Measurements ==
  Mux : Mux  Inputs=1
  Mux3 : Mux
  Machines Measurements : Outport
  wires:
  Mux3/1 -> Mux/1
  [Wm_G10] -> Mux3/4
  [Q_G10] -> Mux3/3
  [P_G10] -> Mux3/2
  [V_G10] -> Mux3/1
  Mux/1 -> Machines Measurements/1

== system model_T_PSH_IEEE39/SS_NorthSystem2/Subsystem ==
  I_RMS_T (A) : Scope
  P_T (pu) : Scope
  "Power (3ph, Instantaneous)" : powerlib_meascontrol/Measurements/Power (3ph, Instantaneous)
  Q_T(pu) : Scope
  RMS : powerlib_meascontrol/Measurements/RMS  TrueRMS=off  Freq=60  RMSInit=1  Ts=Ts
  RMS1 : powerlib_meascontrol/Measurements/RMS  TrueRMS=off  Freq=60  RMSInit=1  Ts=Ts
  Three-Phase V-I Measurement : powerlib/Measurements/Three-Phase V-I Measurement  VoltageMeasurement=phase-to-phase  SetLabelV=off  LabelV=Vabc  Vpu=off  VpuLL=off  CurrentMeasurement=yes  SetLabelI=off  LabelI=Iabc  Ipu=off  Pbase=100e6  Vbase=500e3  OutputType=Complex  PhasorSimulation=off  PSBequivalent=0
  Three-Phase V-I Measurement1 : powerlib/Measurements/Three-Phase V-I Measurement  VoltageMeasurement=phase-to-ground  SetLabelV=off  LabelV=Vabc  Vpu=off  VpuLL=off  CurrentMeasurement=yes  SetLabelI=off  LabelI=Iabc  Ipu=off  Pbase=100e6  Vbase=500e3  OutputType=Complex  PhasorSimulation=off  PSBequivalent=0
  V_RMS_T (ph-ph) (V) : Scope
  a : PMIOPort  Side=Right
  A : PMIOPort  Port=2  Side=Left
  b : PMIOPort  Port=3  Side=Right
  B : PMIOPort  Port=4  Side=Left
  c : PMIOPort  Port=5  Side=Right
  C : PMIOPort  Port=6  Side=Left
  Out1 : Outport
  Out2 : Outport  Port=2
  Out3 : Outport  Port=3
  Out4 : Outport  Port=4
  wires:
  Three-Phase V-I Measurement1/1 -> "Power (3ph, Instantaneous)"/1
  Three-Phase V-I Measurement/1 -> RMS/1
  Three-Phase V-I Measurement/2 -> RMS1/1
  RMS1/1 -> I_RMS_T (A)/1, Out4/1
  Three-Phase V-I Measurement1/2 -> "Power (3ph, Instantaneous)"/2
  "Power (3ph, Instantaneous)"/1 -> P_T (pu)/1, Out1/1
  "Power (3ph, Instantaneous)"/2 -> Q_T(pu)/1, Out2/1
  RMS/1 -> V_RMS_T (ph-ph) (V)/1, Out3/1
  connections:
  Three-Phase V-I Measurement1/RConn1 -- Three-Phase V-I Measurement/LConn1
  Three-Phase V-I Measurement1/RConn2 -- Three-Phase V-I Measurement/LConn2
  Three-Phase V-I Measurement1/RConn3 -- Three-Phase V-I Measurement/LConn3
  Three-Phase V-I Measurement/RConn2 -- b/RConn1
  Three-Phase V-I Measurement/RConn3 -- c/RConn1
  Three-Phase V-I Measurement1/LConn1 -- A/RConn1
  Three-Phase V-I Measurement/RConn1 -- a/RConn1
  Three-Phase V-I Measurement1/LConn2 -- B/RConn1
  Three-Phase V-I Measurement1/LConn3 -- C/RConn1

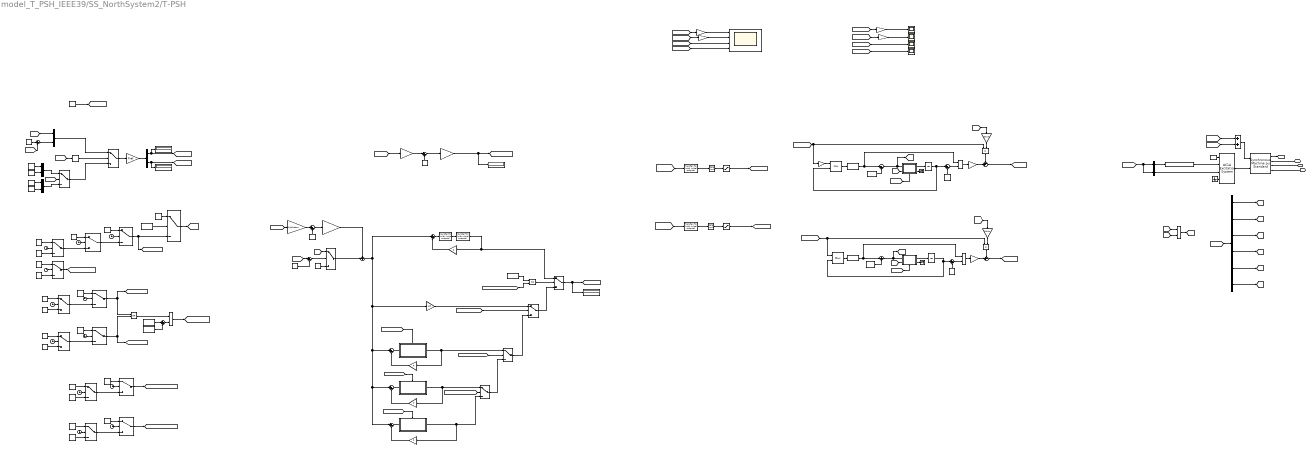
== system model_T_PSH_IEEE39/SS_NorthSystem2/T-PSH ==
  note: Saving routine
  note: Control Center
  note: Generator
  note: Power Distribution
  note: pm_p
  note: pm_t
  note: Turbine mode
  note: Pumping-HSC (Pumping-HSC) transient -> Reach steady state at max speed
  note: h0_t
  note: Pump Gate model (with limiter)
  note: h_t
  note: Turb Gate Reference
  note: Pump model
  note: tmp_t
  note: h_p
  note: pump2hsc
  note: Gen-Pumping (Pumping-Gen) transient -> Reach steady state at max speed
  note: Turbine model
  note: Turb Gate model (with limiter)
  note: Pump Gate Reference
  note: Pref turbine
  note: HSC
  note: tmp_p
  note: hsc2gen
  note: Droop
  note: gen2pump
  note: Mode switching testing
  note: Pump mode
  note: Gen-Pumping (Pumping-Gen) transient -> Reach steady state at max speed
  note: Gen-Pumping (Pumping-Gen) transient -> Reach steady state at max speed
  AC1A Excitation System1 : sps_avr/AC1A Excitation System  Tr=20e-3  KaTa=[400 0.02]  VAminmax=[-14.5 14.5]  VRminmax=[-5.43 6.03]  KfTf=[0.03 1.0]  TbTc=[0 0]  KeTe=[1.0 0.80]  Ve12=[4.18 3.14]  SeVe12=[0.10 0.03]  Kd=0.38  Kc=0.20  v0=[1 1]  TsBlock=0
      settings: SourceProductBaseCode=PS
  Add : Sum
  At : Gain  Gain=At
  At2 : Gain  Gain=At
  Bus Selector2 : BusSelector  OutputSignals="dq0 components.Field current  ifd (pu)"  OutputAsBus=on
  Bus Selector3 : BusSelector  OutputSignals="dq0 components.Stator voltage  vq (pu),dq0 components.Stator voltage  vd (pu),Mechanical.Rotor speed  wm  (pu),Mechanical.Rotor speed deviation  dw (pu),Output active power   Peo (pu),Stator current"
  Bus Selector7 : BusSelector  OutputSignals="dq0 components.Stator voltage  vd (pu),dq0 components.Stator voltage  vq (pu)"  OutputAsBus=on
  Clock{1..12} (12 alike) : Clock
  Constant{1,4..6,9,12,15,17,19..20,24..25,27..28,30} (15 alike) : Constant  Value=0  VectorParams1D=off
  Constant{2..3,7..8,10,16,18,23,26,29,31} (11 alike) : Constant  VectorParams1D=off
  Constant11 : Constant  Value=0.6  VectorParams1D=off
  Constant13 : Constant  Value=Kd  VectorParams1D=off
  Constant14 : Constant  Value=fix_mode  VectorParams1D=off
  Constant21 : Constant  Value=fix_mode  VectorParams1D=off
  Constant22 : Constant  Value=fix_mode  VectorParams1D=off
  Demux : Demux  Outputs=2
  Display{1,9,13..14} (4 alike) : Display
  Divide : Product  Inputs=*/
  Dturb : Gain  Gain=Dturb
  Dturb2 : Gain  Gain=Dturb
  Fcn : Fcn  Expr=(u(2)/u(1))^2
  Fcn1 : Fcn  Expr=(u(2)/u(1))^2
  Fcn3 : Fcn  Expr=sqrt(u(1)^2 + u(2)^2)
  Gain : Gain  Gain=1/At/Hdam
  Gain1 : Gain  Gain=1/sqrt(Hdam)
  Gain2 : Gain  Gain=Pref
  Gain3 : Gain  Gain=1/At/Hdam
  Gain4 : Gain  Gain=R/sqrt(Hdam)
  Gain5 : Gain  Gain=-1
  Gain{6..9} (4 alike) : Gain  Gain=Sn/1e6
  Ground2 : Ground
  Hdam : Constant  Value=Hdam
  Hdam2 : Constant  Value=Hdam
  Integrator3 : Integrator  InitialCondition=pgen_turb/At/Hdam +qNL
  Integrator4 : Integrator  InitialCondition=-1*(pgen_pump/At/Hdam +qNL)
  Interval Test : simulink/Logic and Bit Operations/Interval Test  IntervalClosedRight=off  uplimit=1  IntervalClosedLeft=off  lowlimit=0.5  OutDataTypeStr=boolean
  Logical Operator : Logic  Operator=OR  AllPortsSameDT=off  OutDataTypeStr=boolean
  Logical Operator1 : Logic  Operator=OR  AllPortsSameDT=off  OutDataTypeStr=boolean
  Mux{,1..4} (5 alike) : Mux  Inputs=2
      Mux3 settings: DisplayOption=signals
      Mux4 settings: DisplayOption=signals
  Pmech_pump : Scope
  Pmech_turb : Scope
  Product{,1,3..5} (5 alike) : Product
  Pump_gate_value : Scope
  R{,2..4} (4 alike) : Gain  Gain=R
  R1 : Gain  Gain=1/R
  Rate Limiter2 : RateLimiter  RisingSlewLimit=Velm  FallingSlewLimit=-Velm  SampleTimeMode=inherited
  Rate Limiter3 : RateLimiter  RisingSlewLimit=Velm  FallingSlewLimit=-Velm  SampleTimeMode=inherited
  Resettable Subsystem : Subsystem  TreatAsAtomicUnit=on
  Resettable Subsystem1 : Subsystem  TreatAsAtomicUnit=on
  Resettable Subsystem2 : Subsystem  TreatAsAtomicUnit=on
  Saturation5 : Saturate  UpperLimit=Gmax  LowerLimit=Gmin
  Saturation6 : Saturate  UpperLimit=Gmax  LowerLimit=Gmin
  Scope3 : Scope  NumInputPorts=4
  Subsystem : Subsystem
      settings: PortSchema="{\"entries\":[{\"content\":{\"sides\":[{\"content\":{\"connectorIds\":[\"In1\",\"In2\"]},\"type\":\"ConnectorPlacement.EquallySpacedRectSide\",\"uuid\":\"6eb046cc-a875-4440-962f-cbe88b973247\"},{\"content\":{\"connectorIds\":[\"Out1\",\"Out2\"],\"side\":\"RIGHT\"},\"type\":\"ConnectorPlacement.EquallySpacedRectSide\",\"uuid\":\"6c4547ca-5e48-4232-bd1a-e4a1f21ddf27\"},{\"content\":{\"connectorIds\":[],\"side\":\"TOP\"},\"type\":\"ConnectorPlacement.EquallySpacedRectSide\",\"uuid\":\"73afd8ec-eaec-49a9-81eb-ba5265f116ea\"},{\"content\":{\"connectorIds\":[\"In3\"],\"side\":\"BOTTOM\"},\"type\":\"ConnectorPlacement.EquallySpacedRectSide\",\"uuid\":\"d8a51b86-ed5e-437a-832f-dcb2679a64da\"},{\"content\":{\"connectorIds\":[],\"side\":\"HIDDEN\"},\"type\":\"ConnectorPlacement.EquallySpacedRectSide\",\"uuid\":\"6bd0488f-5829-4a81-83be-3e4f1bfc098c\"}]},\"type\":\"ConnectorPlacement.EquallySpacedConnector\",\"uuid\":\"9f8fbde0-4909-466c-8af4-dc3b94617a86\"}],\"packageUris\":[\"http://schema.mathworks.com/mf0/Connector/R2020b\"],\"version\":\"1.0\"}"
  Subsystem1 : Subsystem
      settings: PortSchema="{\"entries\":[{\"content\":{\"sides\":[{\"content\":{\"connectorIds\":[\"In1\",\"In2\"]},\"type\":\"ConnectorPlacement.EquallySpacedRectSide\",\"uuid\":\"6eb046cc-a875-4440-962f-cbe88b973247\"},{\"content\":{\"connectorIds\":[\"Out1\",\"Out2\"],\"side\":\"RIGHT\"},\"type\":\"ConnectorPlacement.EquallySpacedRectSide\",\"uuid\":\"6c4547ca-5e48-4232-bd1a-e4a1f21ddf27\"},{\"content\":{\"connectorIds\":[],\"side\":\"TOP\"},\"type\":\"ConnectorPlacement.EquallySpacedRectSide\",\"uuid\":\"73afd8ec-eaec-49a9-81eb-ba5265f116ea\"},{\"content\":{\"connectorIds\":[\"In3\"],\"side\":\"BOTTOM\"},\"type\":\"ConnectorPlacement.EquallySpacedRectSide\",\"uuid\":\"7cadaec1-3498-40ee-964f-8acc3835796a\"},{\"content\":{\"connectorIds\":[],\"side\":\"HIDDEN\"},\"type\":\"ConnectorPlacement.EquallySpacedRectSide\",\"uuid\":\"6bd0488f-5829-4a81-83be-3e4f1bfc098c\"}]},\"type\":\"ConnectorPlacement.EquallySpacedConnector\",\"uuid\":\"9f8fbde0-4909-466c-8af4-dc3b94617a86\"}],\"packageUris\":[\"http://schema.mathworks.com/mf0/Connector/R2020b\"],\"version\":\"1.0\"}"
  Sum : Sum  Inputs=+-|
  Sum{1,4..5,7..8,11,13..15} (9 alike) : Sum  Inputs=|+-
  Sum10 : Sum  Inputs=|-+
  Sum12 : Sum  Inputs=-+|
  Sum2 : Sum  Inputs=|-+
  Sum3 : Sum  Inputs=|++
  Sum6 : Sum  Inputs=-+|
  Sum9 : Sum  Inputs=|++
  Switch1 : Switch  Criteria=u2 > Threshold  Threshold=t_hsc2gen
  Switch10 : Switch  Criteria=u2 ~= 0  Threshold=1
  Switch11 : Switch  Criteria=u2 > Threshold  Threshold=t_pump2hsc
  Switch12 : Switch  Criteria=u2 > Threshold  Threshold=t_pump2hsc + max_delay_pump2hsc
  Switch{9,13..15} (4 alike) : Switch  Threshold=1  ZeroCross=off
  Switch16 : Switch  Criteria=u2 > Threshold  Threshold=t_gen2pump
  Switch17 : Switch  Criteria=u2 > Threshold  Threshold="t_gen2pump  + max_delay_gen2pump"
  Switch18 : Switch  Criteria=u2 > Threshold  Threshold=t_pump2hsc
  Switch19 : Switch  Criteria=u2 > Threshold  Threshold=t_pump2hsc + max_delay_pump2hsc
  Switch2 : Switch  Criteria=u2 > Threshold  Threshold=t_gen2pump
  Switch20 : Switch  Criteria=u2 > Threshold  Threshold=t_hsc2gen
  Switch3 : Switch  Criteria=u2 > Threshold  Threshold=1
  Switch4 : Switch  Criteria=u2 ~= 0  Threshold=1
  Switch5 : Switch  Criteria=u2 > Threshold  Threshold=t_pump2hsc
  Switch6 : Switch  Threshold=1
  Switch7 : Switch  Criteria=u2 > Threshold  Threshold=t_gen2pump
  Switch8 : Switch  Criteria=u2 > Threshold  Threshold="t_gen2pump  + max_delay_gen2pump"
  Synchronous Machine pu Standard : powerlib/Machines/Synchronous Machine pu Standard  PresetModel=No  MechanicalLoad=Mechanical power Pm  ShowDetailedParameters=on  RotorType=Salient-pole  Units=per unit standard parameters  MeasurementBus=off  NominalParameters=[ Sn Vn 60]  Reactances1=[ 1.81, 0.3, 0.23, 1.76, 0.65, 0.25, 0.15 ]  Reactances2="[ 0.92, 0.169, 0.135, 0.510, 0.2,  0.13]"  dAxisTimeConstants=Short-circuit  qAxisTimeConstants=Open-circuit  TimeConstants1="[ 4.4849  0.0681  0.1  ]"  TimeConstants2=[ 8.0, 0.03, 1.0, 0.07 ]  TimeConstants3="[  4.49  0.0681  0.0513  ]"  TimeConstants4=[ 8.0, 0.03, 0.3371, 0.0295 ]  TimeConstants5=[ 4.3, 0.032, 0.05 ]  TimeConstants6=[ 1.3201, 0.023, 1.0, 0.07 ]  TimeConstants7=[0.012 0.003 0.003]  TimeConstants8=[ 1.3201, 0.0231, 0.3371, 0.0295 ]  StatorResistance=2.8544e-3  Mechanical=[ 6 0 2]  PolePairs=20  InitialConditions=[0 -94.2826 0.750185 0.750185 0.750185 -24.943 -144.943 95.057 1.29071]  SetSaturation=off  Saturation=[0.6404,0.7127,0.8441,0.9214,0.9956,1.082,1.19,1.316,1.457;0.7,0.7698,0.8872,0.9466,0.9969,1.046,1.1,1.151,1.201]  LoadFlowParameters=[1,0,0,0,0]  TsPowergui=0  TsBlock=-1  IterativeModel=Trapezoidal non iterative  IterativeDiscreteModel=Trapezoidal non iterative  BusType=PV  Pref=0  Qref=0  Qmin=-inf  Qmax=inf  PLF=0  QLF=0
  Terminator : Terminator
  Terminator1 : Terminator
  Transfer Fcn (with initial outputs)1 : simulink_extras/Additional Linear/Transfer Fcn (with initial outputs)  N=[1]  D="[Tg  1]"  Y0=(pgen_pump/At/Hdam +qNL)/sqrt(Hdam)  U0=0
  Transfer Fcn (with initial outputs)2 : simulink_extras/Additional Linear/Transfer Fcn (with initial outputs)  N=[1]  D="[Tg  1]"  Y0=(pgen_turb/At/Hdam +qNL)/sqrt(Hdam)  U0=0
  Transfer Fcn (with initial outputs)4 : simulink_extras/Additional Linear/Transfer Fcn (with initial outputs)  N=[1]  D="[Tf  1]"  Y0=0  U0=0
  Transfer Fcn (with initial outputs)5 : simulink_extras/Additional Linear/Transfer Fcn (with initial outputs)  N=[Tr 1]  D="[Tr*r  0]"  Y0=(pgen_turb/At/Hdam +qNL)/sqrt(Hdam)  U0=0
  Turb_gate_value : Scope
  Vref2 : Constant  Value=1.01
  qNL : Constant  Value=-qNL
  qNL1 : Constant  Value=qNL
  qNL2 : Constant  Value=qNL
  qNL3 : Constant  Value=qNL
  A1 : PMIOPort  Side=Right
  B1 : PMIOPort  Port=2  Side=Right
  C1 : PMIOPort  Port=3  Side=Right
  wires:
  Bus Selector3/4 -> [Dw]  "<Rotor speed deviation  dw (pu)>"
  [w] -> Divide/2
  Fcn3/1 -> AC1A Excitation System1/2  "Vt"
  [Peo] -> Divide/1
  [Pmech_pump] -> Add/1
  Divide/1 -> [Te]
  Bus Selector3/1 -> [Vdq]  "<Stator voltage  vq (pu)>"
  Bus Selector3/2 -> [Vds]  "<Stator voltage  vd (pu)>"
  Bus Selector3/3 -> [w]  "<Rotor speed  wm  (pu)>"
  Synchronous Machine pu Standard/1 -> [m]
  [m] -> Bus Selector2/1, Bus Selector7/1
  [Pmech_turb] -> Add/2
  Ground2/1 -> AC1A Excitation System1/4
  Bus Selector7/1 -> Fcn3/1  "Vd Vq"
  Bus Selector3/6 -> [Iabc]  "<Stator current>"
  Vref2/1 -> AC1A Excitation System1/1
  Bus Selector3/5 -> [Peo]  "<Output active power   Peo (pu)>"
  Add/1 -> Synchronous Machine pu Standard/1
  Bus Selector2/1 -> AC1A Excitation System1/3  "Ifd"
  [m] -> Bus Selector3/1
  AC1A Excitation System1/1 -> Synchronous Machine pu Standard/2
  Gain3/1 -> Sum9/1
  Sum2/1 -> [h_p], Subsystem/1(h_p)
  At/1 -> Sum6/2
  [h_t] -> Subsystem/2(h_t)
  Integrator4/1 -> Sum4/1, Mux3/2
  [Kd_flag] -> Switch4/2
  [Kd_flag] -> Interval Test/1
  Constant4/1 -> Mux/2
  Gain/1 -> Sum3/1
  Transfer Fcn (with initial outputs)1/1 -> Rate Limiter3/1
  Saturation5/1 -> [Turb_gate_value]
  [Pump_gate_value] -> Scope3/3
  [Pmech_turb] -> Gain7/1
  Transfer Fcn (with initial outputs)2/1 -> Rate Limiter2/1
  [Turb_gate_value] -> Scope3/4
  Rate Limiter2/1 -> Saturation5/1
  Constant20/1 -> [share_flag]
  Clock1/1 -> Switch5/2
  Product/1 -> At/1
  Constant15/1 -> Switch10/3
  Sum14/1 -> Switch10/2
  Subsystem/1(q_pump) -> Integrator4/1
  [Dw] -> Switch10/1
  Transfer Fcn (with initial outputs)5/1 -> Switch13/1, R/1
  Constant16/1 -> Sum14/2
  R/1 -> Sum15/2
  Sum11/1 -> Product4/2
  Constant7/1 -> Mux2/2
  Dturb2/1 -> Product5/2
  Clock4/1 -> Switch8/2
  Switch5/1 -> Switch1/3
  Constant8/1 -> Switch7/1
  [share_flag] -> Subsystem1/3(In1)
  Sum15/1 -> Transfer Fcn (with initial outputs)4/1
  [Pset_turb] -> Gain3/1
  [Kd_flag] -> Sum13/2
  Clock3/1 -> Switch2/2
  Switch2/1 -> Switch5/3
  [h_p] -> Subsystem1/2(h_p)
  Dturb/1 -> Product3/2
  Fcn1/1 -> Sum10/1, Product4/1
  Product4/1 -> At2/1
  Sum9/1 -> Gain4/1
  [Dw] -> Dturb2/1
  [Turb_gate_value] -> Product5/1, Mux4/1
  Integrator3/1 -> Sum11/1, Mux4/2
  Sum10/1 -> Subsystem1/1(h_t), [h_t]
  Hdam2/1 -> Sum10/2
  At2/1 -> Sum12/2
  Constant9/1 -> Switch8/1
  Constant12/1 -> Switch1/1
  Rate Limiter3/1 -> Saturation6/1
  [Turb_gate_ref] -> Transfer Fcn (with initial outputs)2/1
  Mux2/1 -> Switch4/3
  Resettable Subsystem/1(Out1) -> Switch14/1, R2/1
  Switch1/1 -> [neg_hsc2gen_flag], Switch6/3
  Constant1/1 -> Switch2/3
  Clock12/1 -> Switch20/2
  Logical Operator1/1 -> Switch13/2
  Constant31/1 -> Sum8/1
  Constant2/1 -> Sum13/1
  Switch20/1 -> [after_clutch_pump2hsc_flag]
  Subsystem1/1(q_turb) -> Integrator3/1
  Mux1/1 -> Switch3/1
  [Pump_gate_ref] -> Transfer Fcn (with initial outputs)1/1
  Constant21/1 -> Sum8/2
  Clock8/1 -> Switch16/2
  Constant23/1 -> Switch16/3
  Subsystem1/2(q_pump) -> Terminator1/1
  Switch19/1 -> Switch20/3
  Constant13/1 -> Switch6/1
  [fast_transient_flag] -> Switch9/2
  Constant5/1 -> Switch7/3
  Switch14/1 -> Switch9/3
  Gain6/1 -> Scope3/1
  Sum4/1 -> Product/2
  [mode_switching_initialization] -> Logical Operator1/2
  Switch7/1 -> Switch8/3
  [Kd_flag] -> Sum14/1
  Clock6/1 -> Switch12/2
  Constant14/1 -> Switch6/2
  Clock11/1 -> Switch19/2
  Mux/1 -> Switch4/1
  R4/1 -> Sum7/2
  Sum6/1 -> [Pmech_pump]
  Clock9/1 -> Switch18/2
  [after_clutch_pump2hsc_flag] -> Switch15/2
  Demux/1 -> [Pset_pump], Display13/1
  qNL/1 -> Sum4/2
  Switch9/1 -> Switch13/3
  qNL2/1 -> Sum11/2
  Sum13/1 -> Mux1/2
  Constant28/1 -> Switch19/3
  Constant30/1 -> Switch20/1
  Constant27/1 -> Switch18/1
  Constant26/1 -> Switch17/1
  Constant29/1 -> Switch19/1
  [after_clutch_gen2pump_flag] -> Switch14/2
  Switch3/1 -> Gain2/1
  Constant19/1 -> Switch12/1
  Transfer Fcn (with initial outputs)4/1 -> Transfer Fcn (with initial outputs)5/1
  Switch18/1 -> [after_clutch_gen2pump_flag]
  Gain2/1 -> Demux/1
  Clock10/1 -> Switch17/2
  Switch11/1 -> Switch12/3
  Constant3/1 -> Mux/1
  R2/1 -> Sum1/2
  Switch17/1 -> Switch18/3
  [neg_hsc2gen_flag] -> Resettable Subsystem2/Reset
  Switch16/1 -> [mode_switching_initialization]
  Switch8/1 -> Logical Operator/1, [neg_gen2pump_flag]
  Sum8/1 -> Product1/2
  Constant25/1 -> Switch17/3
  Product1/1 -> [fast_transient_flag]
  Saturation6/1 -> [Pump_gate_value]
  Constant24/1 -> Switch16/1
  Constant6/1 -> Mux2/1
  Product5/1 -> Sum12/1
  [neg_pump2hsc_flag] -> Resettable Subsystem1/Reset
  R1/1 -> Switch9/1
  Constant22/1 -> Logical Operator1/1
  Switch6/1 -> [Kd_flag]
  [Kd_flag] -> Mux1/1
  Constant10/1 -> Switch2/1
  Switch10/1 -> Sum/2
  Resettable Subsystem2/1(Out1) -> Switch15/3, R4/1
  Switch15/1 -> Switch14/3
  Sum12/1 -> [Pmech_turb]
  Fcn/1 -> Sum2/1, Product/1
  [Pmech_pump] -> Gain6/1
  Resettable Subsystem1/1(Out1) -> Switch15/1, R3/1
  Product3/1 -> Sum6/1
  Sum7/1 -> Resettable Subsystem2/1(In1)
  Sum1/1 -> Resettable Subsystem/1(In1)
  Switch13/1 -> Display1/1, [Turb_gate_ref]
  Sum5/1 -> Resettable Subsystem1/1(In1)
  Subsystem/2(q_turb) -> Terminator/1
  R3/1 -> Sum5/2
  Clock5/1 -> Switch7/2
  [neg_gen2pump_flag] -> Resettable Subsystem/Reset
  Demux/2 -> [Pset_turb], Display14/1
  [share_flag] -> Subsystem/3(In1)
  Mux4/1 -> Fcn1/1
  Clock2/1 -> Switch1/2
  Sum/1 -> Sum7/1, Sum5/1, Sum1/1, R1/1, Sum15/1
  Hdam/1 -> Sum2/2
  Constant18/1 -> Switch11/1
  Gain4/1 -> Sum/1
  Switch12/1 -> [neg_pump2hsc_flag], Logical Operator/2
  Interval Test/1 -> Switch3/2
  Sum3/1 -> Gain1/1
  Gain7/1 -> Scope3/2
  Mux3/1 -> Fcn/1
  Constant17/1 -> Switch11/3
  Clock7/1 -> Switch11/2
  qNL1/1 -> Sum3/2
  Switch4/1 -> Switch3/3
  Gain1/1 -> Display9/1, [Pump_gate_ref]
  [Dw] -> Dturb/1
  [Pump_gate_value] -> Product3/1, Gain5/1
  qNL3/1 -> Sum9/2
  Logical Operator/1 -> Product1/1
  Constant11/1 -> Switch5/1
  [Pset_pump] -> Gain/1
  Gain5/1 -> Mux3/1
  [Pmech_pump] -> Gain8/1
  Gain8/1 -> Pmech_pump/1
  [Pmech_turb] -> Gain9/1
  [Pump_gate_value] -> Pump_gate_value/1
  Gain9/1 -> Pmech_turb/1
  [Turb_gate_value] -> Turb_gate_value/1
  connections:
  Synchronous Machine pu Standard/RConn3 -- C1/RConn1
  Synchronous Machine pu Standard/RConn2 -- B1/RConn1
  Synchronous Machine pu Standard/RConn1 -- A1/RConn1

== system model_T_PSH_IEEE39/SS_WestSystem1/Buses Current_W ==
  Mux3 : Mux  Inputs=5
  Current : Outport
  wires:
  Mux3/1 -> Current/1
  [I_L4] -> Mux3/1
  [I_bus_5] -> Mux3/2
  [I_L8] -> Mux3/3
  [I_bus_9] -> Mux3/4
  [I_L39] -> Mux3/5

== system model_T_PSH_IEEE39/SS_WestSystem1/Buses voltages_W ==
  Mux3 : Mux  Inputs=5
  Voltages : Outport
  wires:
  [V_L39] -> Mux3/5
  [V_bus_9] -> Mux3/4
  [V_L8] -> Mux3/3
  [V_bus_5] -> Mux3/2
  [V_L4] -> Mux3/1
  Mux3/1 -> Voltages/1
